simulink subsystem "qep_algorithm"  (R2025b)
settings: Solver=VariableStepAuto  StartTime=0.0  StopTime=10.0  RelTol=1e-3
values from neighbouring files (symbols this model uses):
  dataType = 'single'    [mcb_pmsm_foc_f280049C_data.m]    (also in mcb_pmsm_foc_f28335_data.m; mcb_pmsm_foc_qep_f28035_data.m = fixdt(1,32,17))
  inverter = mcb.getInverterParameters('BoostXL-DRV8305')    [mcb_pmsm_foc_f280049C_data.m]    (also in mcb_pmsm_foc_f28335_data.m = mcb.getInverterParameters('DRV8312-C2-KIT'); mcb_pmsm_foc_qep_f28035_data.m = mcb.getInverterParameters('DRV8312-C2-KIT'))
  pmsm = mcb.getPMSMParameters('BLY171D')    [mcb_pmsm_foc_f280049C_data.m]    (also in mcb_pmsm_foc_f28335_data.m; mcb_pmsm_foc_qep_f28035_data.m)
  PU_System = mcb.getPUSystemParameters(pmsm,inverter)    [mcb_pmsm_foc_f280049C_data.m]    (also in mcb_pmsm_foc_f28335_data.m; mcb_pmsm_foc_qep_f28035_data.m)
  target = mcb.getProcessorParameters('F280049C',PWM_frequency)    [mcb_pmsm_foc_f280049C_data.m]    (also in mcb_pmsm_foc_f28335_data.m = mcb.getProcessorParameters('F28335',PWM_frequency); mcb_pmsm_foc_qep_f28035_data.m = mcb.getProcessorParameters('F28035',PWM_frequency))
libraries: mcbpositiondecoderlib x3, simulink x2, mcbcontrolslib x1

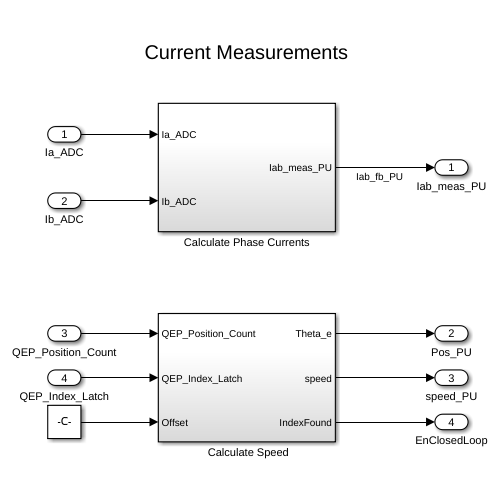
[thumbnail: Simulink's stored preview of the top-level diagram]
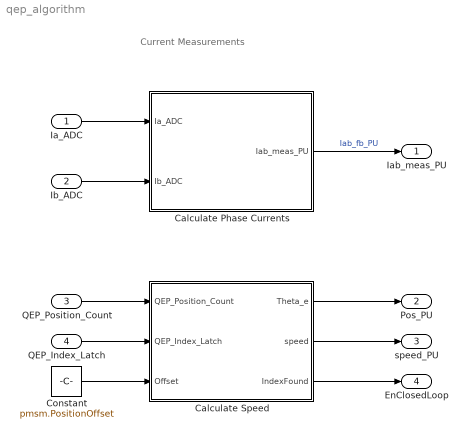
== system qep_algorithm ==
  note: Current Measurements
  Ia_ADC : Inport
  Ib_ADC : Inport  Port=2
  QEP_Position_Count : Inport  Port=3
  QEP_Index_Latch : Inport  Port=4
  " Calculate Speed" : Subsystem
  Calculate Phase Currents : Subsystem
  Constant : Constant  Value=pmsm.PositionOffset  SampleTime=-1
  Iab_meas_PU : Outport
  Pos_PU : Outport  Port=2
  speed_PU : Outport  Port=3
  EnClosedLoop : Outport  Port=4
  wires:
  " Calculate Speed"/2(speed) -> speed_PU/1
  Calculate Phase Currents/1(Iab_meas_PU) -> Iab_meas_PU/1  "Iab_fb_PU"
  QEP_Position_Count/1 -> " Calculate Speed"/1(QEP_Position_Count)
  " Calculate Speed"/1(Theta_e) -> Pos_PU/1
  Ia_ADC/1 -> Calculate Phase Currents/1(Ia_ADC)
  Ib_ADC/1 -> Calculate Phase Currents/2(Ib_ADC)
  Constant/1 -> " Calculate Speed"/3(Offset)
  QEP_Index_Latch/1 -> " Calculate Speed"/2(QEP_Index_Latch)
  " Calculate Speed"/3(IndexFound) -> EnClosedLoop/1

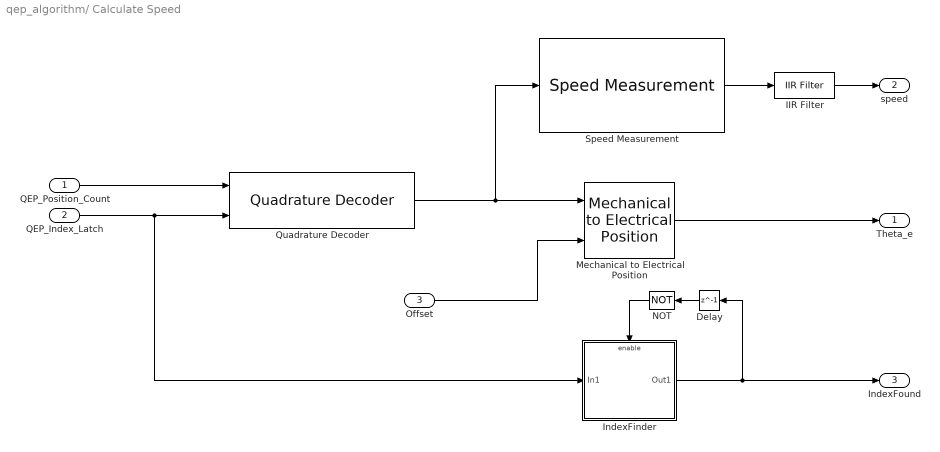
== system qep_algorithm/ Calculate Speed ==
  QEP_Position_Count : Inport
  QEP_Index_Latch : Inport  Port=2
  Offset : Inport  Port=3
  Delay : Delay  DelayLength=1
  IIR Filter : mcbcontrolslib/IIR Filter  VariantControl=Low Pass Filter  VariantSelect=Low-pass  FilterConstantInputType=Specify via dialog  Filter_constant=0.01  InitialOutput=Specify via dialog  InitialOutputValue=0  ExternalReset=none  advancedSettings=off  Ts=50e-6  cutOff_freq=32.1525
  IndexFinder : Subsystem
  Mechanical to Electrical Position : mcbpositiondecoderlib/Mechanical to Electrical Position  PolePairsInputType=Specify via dialog  NrPP=pmsm.p  selectedRange=Per unit  MechOfstInputType=Input port  mechOffsetIn=0  maxAngleIn=1  InputDataType=dataType  VariantSelect=floating-point
  NOT : Logic  Operator=NOT  AllPortsSameDT=off  OutDataTypeStr=boolean
  Quadrature Decoder : mcbpositiondecoderlib/Quadrature Decoder  ParameterInputType=off  CountsPerRevInverseDataType=single  EncoderSlitsPerRevolution=pmsm.QEPSlits  EncoderCountsPerSlit=4  CounterSize=16 bits  ExternalIndexCount=on  PositionUnit=Per unit  PositionDataType=dataType
  Speed Measurement : mcbpositiondecoderlib/Speed Measurement  DiscreteStepInput=off  LastDiscreteStepInput=off  PositionUnit=Per unit  PositionScalingDatatype=uint32  SpeedCalculationMode=Time interval for speed calculation  TempSpeedCalculationMode=Time interval for speed calculation  SampleTimeAsync=Ts  MaximumApplicationSpeed=6000  SpeedResolution=5e-6  DelayLength=20  MaximumMeasurableSpeed=29999  MeasurableSpeedResolution=1.397e-05  SpeedUnit=Per unit based on dialog  TempSpeedUnit=RPM  PerUnitSpeed=PU_System.N_base  SpeedDataType=dataType
  Theta_e : Outport  VectorParamsAs1DForOutWhenUnconnected=off
  speed : Outport  Port=2  VectorParamsAs1DForOutWhenUnconnected=off
  IndexFound : Outport  Port=3  InitialOutput=0  VectorParamsAs1DForOutWhenUnconnected=off
  wires:
  Delay/1 -> NOT/1
  QEP_Index_Latch/1 -> Quadrature Decoder/2, IndexFinder/1(In1)
  IndexFinder/1(Out1) -> IndexFound/1, Delay/1
  NOT/1 -> IndexFinder/Enable
  IIR Filter/1 -> speed/1
  Offset/1 -> Mechanical to Electrical Position/2
  QEP_Position_Count/1 -> Quadrature Decoder/1
  Quadrature Decoder/1 -> Mechanical to Electrical Position/1, Speed Measurement/1
  Speed Measurement/1 -> IIR Filter/1
  Mechanical to Electrical Position/1 -> Theta_e/1

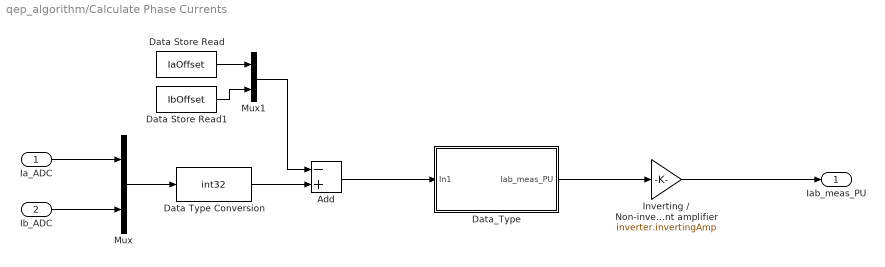
== system qep_algorithm/Calculate Phase Currents ==
  Ia_ADC : Inport
  Ib_ADC : Inport  Port=2
  Add : Sum  Inputs=-+
  Data Store Read : DataStoreRead  DataStoreName=IaOffset  IndexOptions=Index vector (dialog)  Indices=1  OutputSizes=1
  Data Store Read1 : DataStoreRead  DataStoreName=IbOffset  IndexOptions=Index vector (dialog)  Indices=1  OutputSizes=1
  Data Type Conversion : DataTypeConversion  OutDataTypeStr=int32  ConvertRealWorld=Stored Integer (SI)  SaturateOnIntegerOverflow=off  RndMeth=Floor
  Data_Type : Subsystem  Variant=on
  Inverting / Non-inverting Current measurement amplifier : Gain  Gain=inverter.invertingAmp  RndMeth=Simplest  OutDataTypeStr=Inherit: Same as input
  Mux : Mux  Inputs=2
  Mux1 : Mux  Inputs=2
  Iab_meas_PU : Outport  VectorParamsAs1DForOutWhenUnconnected=off
  wires:
  Inverting / Non-inverting Current measurement amplifier/1 -> Iab_meas_PU/1
  Data Store Read1/1 -> Mux1/2
  Data Store Read/1 -> Mux1/1
  Data_Type/1(Iab_meas_PU) -> Inverting / Non-inverting Current measurement amplifier/1
  Mux/1 -> Data Type Conversion/1
  Ib_ADC/1 -> Mux/2
  Add/1 -> Data_Type/1(In1)
  Ia_ADC/1 -> Mux/1
  Data Type Conversion/1 -> Add/2
  Mux1/1 -> Add/1

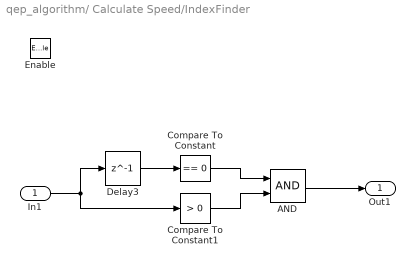
== system qep_algorithm/ Calculate Speed/IndexFinder ==
  In1 : Inport
  Enable : EnablePort
  AND : Logic  AllPortsSameDT=off  OutDataTypeStr=boolean
  Compare To Constant : simulink/Logic and Bit Operations/Compare To Constant  relop===  const=0  OutDataTypeStr=boolean
  Compare To Constant1 : simulink/Logic and Bit Operations/Compare To Constant  relop=>  const=0  OutDataTypeStr=boolean
  Delay3 : Delay  DelayLength=1
  Out1 : Outport
  wires:
  AND/1 -> Out1/1
  Delay3/1 -> Compare To Constant/1
  Compare To Constant/1 -> AND/1
  Compare To Constant1/1 -> AND/2
  In1/1 -> Compare To Constant1/1, Delay3/1

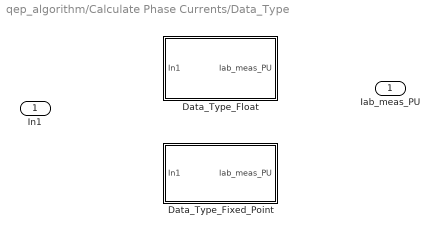
== system qep_algorithm/Calculate Phase Currents/Data_Type ==
  In1 : Inport
  Data_Type_Fixed_Point : Subsystem  VariantControl=~isequal(dataType,'single')
  Data_Type_Float : Subsystem  VariantControl=isequal(dataType,'single')
  Iab_meas_PU : Outport

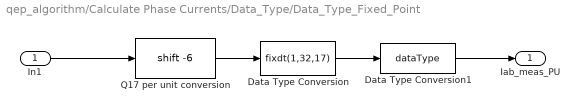
== system qep_algorithm/Calculate Phase Currents/Data_Type/Data_Type_Fixed_Point ==
  In1 : Inport
  Data Type Conversion : DataTypeConversion  OutDataTypeStr=fixdt(1,32,17)  ConvertRealWorld=Stored Integer (SI)  RndMeth=Simplest  SaturateOnIntegerOverflow=off
  Data Type Conversion1 : DataTypeConversion  OutDataTypeStr=dataType  RndMeth=Simplest  SaturateOnIntegerOverflow=off
  Q17 per unit conversion : ArithShift  BitShiftNumber=-6
  Iab_meas_PU : Outport
  wires:
  In1/1 -> Q17 per unit conversion/1
  Data Type Conversion1/1 -> Iab_meas_PU/1
  Data Type Conversion/1 -> Data Type Conversion1/1
  Q17 per unit conversion/1 -> Data Type Conversion/1

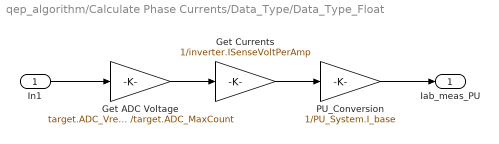
== system qep_algorithm/Calculate Phase Currents/Data_Type/Data_Type_Float ==
  In1 : Inport
  Get ADC Voltage : Gain  Gain=target.ADC_Vref /target.ADC_MaxCount  OutDataTypeStr=dataType  RndMeth=Simplest
  Get Currents : Gain  Gain=1/inverter.ISenseVoltPerAmp  RndMeth=Simplest  OutDataTypeStr=Inherit: Same as input
  PU_Conversion : Gain  Gain=1/PU_System.I_base  RndMeth=Simplest  OutDataTypeStr=Inherit: Same as input
  Iab_meas_PU : Outport
  wires:
  Get ADC Voltage/1 -> Get Currents/1
  Get Currents/1 -> PU_Conversion/1
  PU_Conversion/1 -> Iab_meas_PU/1
  In1/1 -> Get ADC Voltage/1
